simulink model "number_transform_test"  (Simulink 7.6)
settings: Solver=ode45  StartTime=0.0  StopTime=10.0  RelTol=1e-3
settings Model: Creator=jordan  LastModifiedBy=jordan

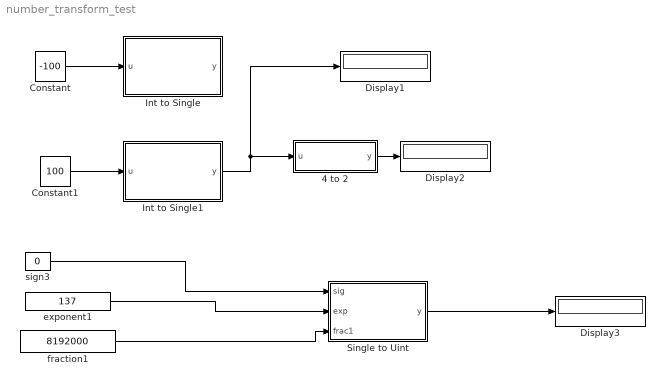
== system number_transform_test ==
  4 to 2 : Stateflow chart  TreatAsAtomicUnit=on
  Constant : Constant  Value=-100  OutDataTypeStr=fixdt(1,14,0)
  Constant1 : Constant  Value=100  OutDataTypeStr=fixdt(0,12,0)
  Display1 : Display
  Display2 : Display
  Display3 : Display
  Int to Single : Stateflow chart  TreatAsAtomicUnit=on
  Int to Single1 : Stateflow chart  TreatAsAtomicUnit=on
  Single to Uint : Stateflow chart  TreatAsAtomicUnit=on
  exponent1 : Constant  Value=137  OutDataTypeStr=uint8
  fraction1 : Constant  Value=8192000  OutDataTypeStr=fixdt(0,24,0)
  sign3 : Constant  Value=0  OutDataTypeStr=uint8
  wires:
  Constant/1 -> Int to Single/1(u)
  4 to 2/1(y) -> Display2/1
  fraction1/1 -> Single to Uint/3(frac1)
  exponent1/1 -> Single to Uint/2(exp)
  sign3/1 -> Single to Uint/1(sig)
  Single to Uint/1(y) -> Display3/1
  Int to Single1/1(y) -> 4 to 2/1(u), Display1/1
  Constant1/1 -> Int to Single1/1(u)

== matlab function Single to Uint ==
  data: sig input uint8; y output fixdt(0,12,0); exp input uint8; frac1 input fixdt(0,24,0)
function y = fcn(sig, exp, frac1)
%#eml

y=fi(0,0,12,0);
z=int16(0);
if (sig==0)
    if (exp>=127)
        buf=uint32(frac1);
        z=int16(exp)-150;
        y=fi(bitshift(buf,z),0,12,0); %-23+(exp-127)
    end
end

== matlab function Int to Single ==
  data: u input fixdt(1,14,0); y output uint32
function y = fcn(u)
%#eml

sig=uint8(0);
exp=uint8(0);
frac=fi(0,0,23,0);

%Transform two's complement integer into unnormalized
%single number
buf=fi(0,1,14,0);
if (u>0)
    sig=uint8(0);
    buf=u;
    frac1=fi(buf,0,23,0);
else
    sig=uint8(1);
    buf=-u;
    frac1=fi(buf,0,23,0);
end

%Normalize floating-point number
buf1=fi(frac1,0,24,0);
p=fi(0,0,5,0);
mask=fi(2^22,0,24,0);
for ind=1:23
    c=bitand(buf1,mask);
    if (c==0)
        buf1=bitshift(buf1,1);
        p=fi(p+1,0,5,0);
    end
end
p=fi(p+1,0,5,0);
buf1=bitshift(fi(frac1,0,24,0),uint8(p));
mask1=fi(2^23-1,0,24,0);
buf1=bitand(buf1,mask1);
frac=fi(buf1,0,23,0);
exp=uint8(127+(22-p));

%Compose floating-point number
z=uint32(0);
if sig
    z=uint32(bitshift(uint32(1),31));
end
buf2=uint32(bitshift(uint32(exp),23));
z=bitor(z,buf2);
z=bitor(z,uint32(frac));
y=z;

== matlab function Int to Single1 ==
  data: u input fixdt(0,12,0); y output uint32
function y = fcn(u)
%#eml

sig=uint8(0);
exp=uint8(0);
frac=fi(0,0,23,0);

%Transform two's complement integer into unnormalized
%single number
buf=fi(0,0,12,0);
sig=uint8(0);
buf=u;
frac1=fi(buf,0,23,0);

%Normalize floating-point number
buf1=fi(frac1,0,24,0);
p=fi(0,0,5,0);
mask=fi(2^22,0,24,0);
for ind=1:23
    c=bitand(buf1,mask);
    if (c==0)
        buf1=bitshift(buf1,1);
        p=fi(p+1,0,5,0);
    end
end
p=fi(p+1,0,5,0);
buf1=bitshift(fi(frac1,0,24,0),uint8(p));
mask1=fi(2^23-1,0,24,0);
buf1=bitand(buf1,mask1);
frac=fi(buf1,0,23,0);
exp=uint8(127+(22-p));

%Compose floating-point number
z=uint32(0);
if sig
    z=uint32(bitshift(uint32(1),31));
end
buf2=uint32(bitshift(uint32(exp),23));
z=bitor(z,buf2);
z=bitor(z,uint32(frac));
y=z;

== matlab function 4 to 2 ==
  data: y output single; u input uint32
function y  = fcn(u)
%#eml
y=typecast(u,'single');
